simulink model "Wing_Aerodynamics"  (R2021b)
settings: Solver=VariableStepAuto  StartTime=0.0  StopTime=10.0  RelTol=1e-3
settings Model: Creator=User  LastModifiedBy=User

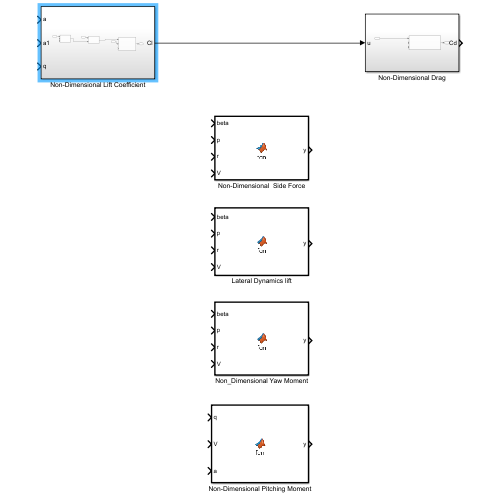
[thumbnail: Simulink's stored preview of the top-level diagram]
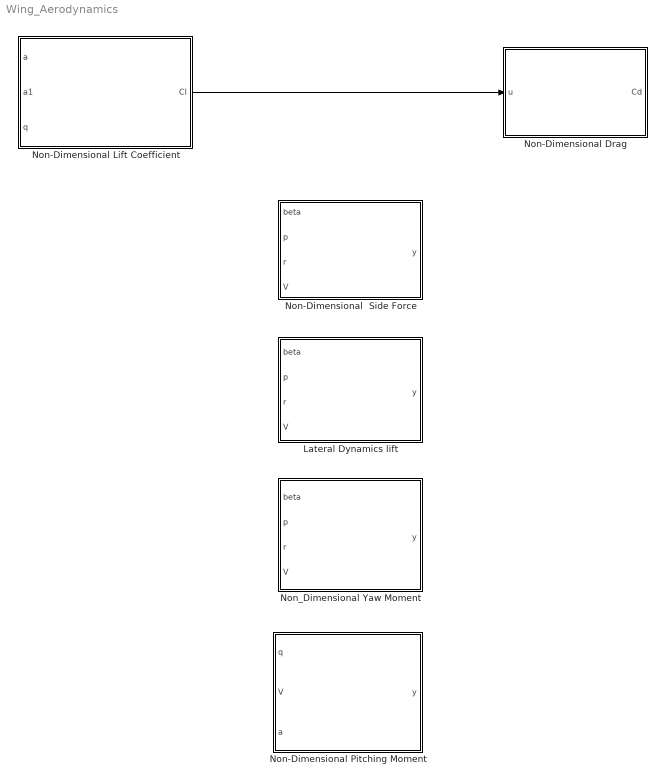
== system Wing_Aerodynamics ==
  Lateral Dynamics lift : MATLAB Function  TreatAsAtomicUnit=on
  Non-Dimensional  Side Force : MATLAB Function  TreatAsAtomicUnit=on
  Non-Dimensional Drag : Subsystem
  Non-Dimensional Lift Coefficient : Subsystem
  Non-Dimensional Pitching Moment : MATLAB Function  TreatAsAtomicUnit=on
  Non_Dimensional Yaw Moment : MATLAB Function  TreatAsAtomicUnit=on
  wires:
  Non-Dimensional Lift Coefficient/1(Cl) -> Non-Dimensional Drag/1(u)

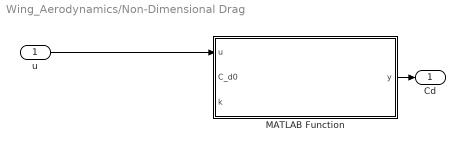
== system Wing_Aerodynamics/Non-Dimensional Drag ==
  u : Inport
  MATLAB Function : MATLAB Function  TreatAsAtomicUnit=on
  Cd : Outport
  wires:
  MATLAB Function/1(y) -> Cd/1
  u/1 -> MATLAB Function/1(u)

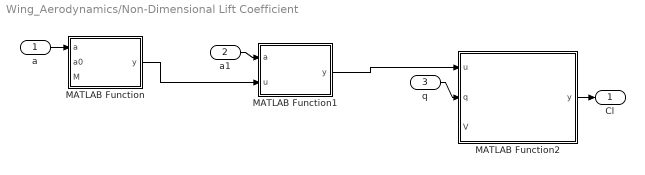
== system Wing_Aerodynamics/Non-Dimensional Lift Coefficient ==
  a : Inport
  a1 : Inport  Port=2
  q : Inport  Port=3
  MATLAB Function : MATLAB Function  TreatAsAtomicUnit=on
  MATLAB Function1 : MATLAB Function  TreatAsAtomicUnit=on
  MATLAB Function2 : MATLAB Function  TreatAsAtomicUnit=on
  Cl : Outport
  wires:
  MATLAB Function/1(y) -> MATLAB Function1/2(u)
  MATLAB Function1/1(y) -> MATLAB Function2/1(u)
  MATLAB Function2/1(y) -> Cl/1
  a1/1 -> MATLAB Function1/1(a)
  q/1 -> MATLAB Function2/2(q)
  a/1 -> MATLAB Function/1(a)

== matlab function Wing_Aerodynamics/Non-Dimensional Lift Coefficient/MATLAB Function1 ==
  data: a input; u input; y output
function y = fcn(a,u)
Cl_0=0.4918;
Cl_a=4.695;
y = (1-u)*(Cl_0+Cl_a*a)+u*(2*sign(a)*power(sin(a),2)*cos(a));

== matlab function Wing_Aerodynamics/Non-Dimensional Lift Coefficient/MATLAB Function ==
  data: a input; y output; a0 input; M input
function y = fcn(a,a0,M)

y = (1+exp(-M(a-a0))+exp(M(a+a0)))/((1+exp(-M(a-a0))*(1+exp(M(a+a0)))));

== matlab function Wing_Aerodynamics/Non-Dimensional Lift Coefficient/MATLAB Function2 ==
  data: u input; y output; q input; V input
function y = fcn(u,q,V)
c=0.39;
C_lq=0;
y = C_lq*(q*c)/(2*V)+u;

== matlab function Wing_Aerodynamics/Non-Dimensional Drag/MATLAB Function ==
  data: u input; y output; C_d0 input; k input
function y = fcn(u,C_d0,k)

y = C_d0+k*u*u;

== matlab function Wing_Aerodynamics/Non-Dimensional  Side Force ==
  data: beta input; y output; p input; r input; V input
function y = fcn(beta,p,r,V)
C_yb=-0.951;
C_yp=0;
C_yr=0.008;
b=2.29;
y = C_yb*beta+C_yp*(p*b)/(2*V)+C_yr*(r*b)/(2*V);

== matlab function Wing_Aerodynamics/Lateral Dynamics lift ==
  data: beta input; y output; p input; r input; V input
function y = fcn(beta,p,r,V)
C_lb=0;
C_lp=-0.43;
C_lr=0.29;
b=2.29;
y = C_lb*beta+C_lp*(p*b)/(2*V)+C_lr*(r*b)/(2*V);

== matlab function Wing_Aerodynamics/Non_Dimensional Yaw Moment ==
  data: beta input; y output; p input; r input; V input
function y = fcn(beta,p,r,V)
C_nb=-0.0812;
C_np=-0.4044;
C_nr==0.05;
b=2.29;
y = C_nb*beta+C_np*(p*b)/(2*V)+C_nr*(r*b)/(2*V);

== matlab function Wing_Aerodynamics/Non-Dimensional Pitching Moment ==
  data: y output; q input; V input; a input
function y  = fcn(q,V,a)
C_m0=-0.0156;
C_ma=0.995;
C_mq=-0.51;
c=0.39;
y = C_m0+C_ma*a+C_mq*(q*c)/(2*V);
